simulink model "untitled"  (Simulink 7.9)
settings: Solver=ode45  StartTime=0.0  StopTime=10.0  RelTol=1e-3
settings Model: Creator=MAR  LastModifiedBy=MAR

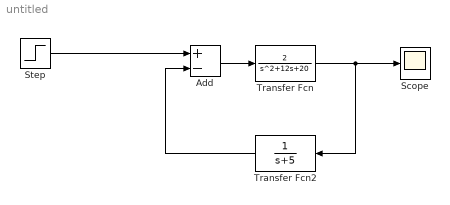
== system untitled ==
  Add : Sum  Inputs=+-
  Scope : Scope
  Step : Step  SampleTime=0
  Transfer Fcn : TransferFcn  Numerator=[2]  Denominator=[1 12 20]
  Transfer Fcn2 : TransferFcn  Numerator=[0 1]  Denominator=[1 5]
  wires:
  Transfer Fcn/1 -> Scope/1, Transfer Fcn2/1
  Add/1 -> Transfer Fcn/1
  Transfer Fcn2/1 -> Add/2
  Step/1 -> Add/1
